simulink subsystem "PTI"  (R2025a)
settings: Solver=VariableStepAuto  StartTime=0.0  StopTime=10.0  RelTol=1e-3
libraries: px4Utilslib x22
settings Model: Creator=gurt1  LastModifiedBy=gurt1

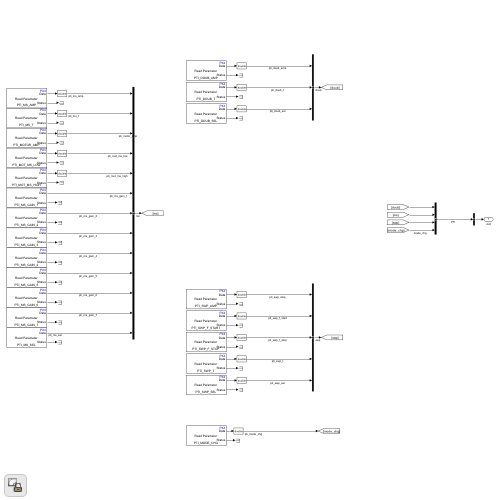
[thumbnail: Simulink's stored preview of the top-level diagram]
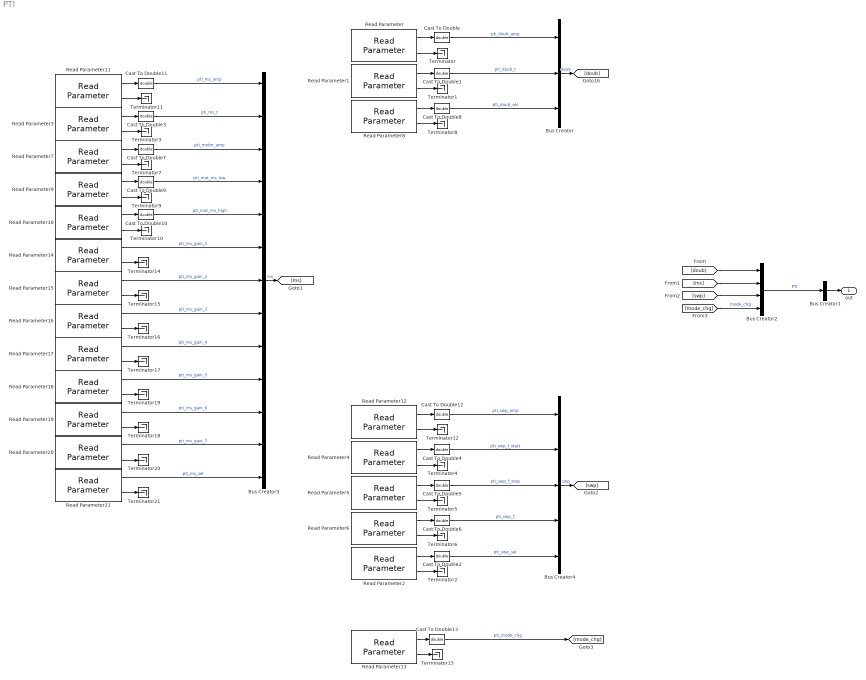
== system PTI ==
  Bus Creator : BusCreator  Inputs=3
  Bus Creator1 : BusCreator  Inputs=1
  Bus Creator2 : BusCreator  Inputs=4
  Bus Creator3 : BusCreator  Inputs=13
  Bus Creator4 : BusCreator  Inputs=5
  Cast To Double{,1..13} (14 alike) : DataTypeConversion  OutDataTypeStr=double  SaturateOnIntegerOverflow=off  RndMeth=Floor
  Read Parameter : px4Utilslib/Read Parameter  ParameterName=PTI_DOUB_AMP  DataType=FLOAT  SampleTime=-1
  Read Parameter1 : px4Utilslib/Read Parameter  ParameterName=PTI_DOUB_T  DataType=FLOAT  SampleTime=-1
  Read Parameter10 : px4Utilslib/Read Parameter  ParameterName=PTI_MOT_MS_HIGH  DataType=FLOAT  SampleTime=-1
  Read Parameter11 : px4Utilslib/Read Parameter  ParameterName=PTI_MS_AMP  DataType=FLOAT  SampleTime=-1
  Read Parameter12 : px4Utilslib/Read Parameter  ParameterName=PTI_SWP_AMP  DataType=FLOAT  SampleTime=-1
  Read Parameter13 : px4Utilslib/Read Parameter  ParameterName=PTI_MODE_CHG  DataType=FLOAT  SampleTime=-1
  Read Parameter14 : px4Utilslib/Read Parameter  ParameterName=PTI_MS_GAIN_1  DataType=FLOAT  SampleTime=-1
  Read Parameter15 : px4Utilslib/Read Parameter  ParameterName=PTI_MS_GAIN_2  DataType=FLOAT  SampleTime=-1
  Read Parameter16 : px4Utilslib/Read Parameter  ParameterName=PTI_MS_GAIN_3  DataType=FLOAT  SampleTime=-1
  Read Parameter17 : px4Utilslib/Read Parameter  ParameterName=PTI_MS_GAIN_4  DataType=FLOAT  SampleTime=-1
  Read Parameter18 : px4Utilslib/Read Parameter  ParameterName=PTI_MS_GAIN_5  DataType=FLOAT  SampleTime=-1
  Read Parameter19 : px4Utilslib/Read Parameter  ParameterName=PTI_MS_GAIN_6  DataType=FLOAT  SampleTime=-1
  Read Parameter2 : px4Utilslib/Read Parameter  ParameterName=PTI_SWP_SEL  DataType=FLOAT  SampleTime=-1
  Read Parameter20 : px4Utilslib/Read Parameter  ParameterName=PTI_MS_GAIN_7  DataType=FLOAT  SampleTime=-1
  Read Parameter21 : px4Utilslib/Read Parameter  ParameterName=PTI_MS_SEL  DataType=FLOAT  SampleTime=-1
  Read Parameter3 : px4Utilslib/Read Parameter  ParameterName=PTI_MS_T  DataType=FLOAT  SampleTime=-1
  Read Parameter4 : px4Utilslib/Read Parameter  ParameterName=PTI_SWP_F_START  DataType=FLOAT  SampleTime=-1
  Read Parameter5 : px4Utilslib/Read Parameter  ParameterName=PTI_SWP_F_STOP  DataType=FLOAT  SampleTime=-1
  Read Parameter6 : px4Utilslib/Read Parameter  ParameterName=PTI_SWP_T  DataType=FLOAT  SampleTime=-1
  Read Parameter7 : px4Utilslib/Read Parameter  ParameterName=PTI_MOTOR_AMP  DataType=FLOAT  SampleTime=-1
  Read Parameter8 : px4Utilslib/Read Parameter  ParameterName=PTI_DOUB_SEL  DataType=FLOAT  SampleTime=-1
  Read Parameter9 : px4Utilslib/Read Parameter  ParameterName=PTI_MOT_MS_LOW  DataType=FLOAT  SampleTime=-1
  Terminator{,1..21} (22 alike) : Terminator
  out : Outport
  wires:
  Read Parameter/2 -> Terminator/1
  Read Parameter/1 -> Cast To Double/1
  Cast To Double/1 -> Bus Creator/1  "pti_doub_amp"
  Bus Creator1/1 -> out/1
  Bus Creator2/1 -> Bus Creator1/1  "PTI"
  Read Parameter1/1 -> Cast To Double1/1
  Read Parameter1/2 -> Terminator1/1
  Cast To Double1/1 -> Bus Creator/2  "pti_doub_t"
  Read Parameter6/2 -> Terminator6/1
  Read Parameter5/2 -> Terminator5/1
  Read Parameter5/1 -> Cast To Double5/1
  Cast To Double6/1 -> Bus Creator4/4  "pti_swp_t"
  Read Parameter6/1 -> Cast To Double6/1
  Read Parameter4/2 -> Terminator4/1
  Read Parameter4/1 -> Cast To Double4/1
  Cast To Double5/1 -> Bus Creator4/3  "pti_swp_f_stop"
  Cast To Double4/1 -> Bus Creator4/2  "pti_swp_f_start"
  Cast To Double11/1 -> Bus Creator3/1  "pti_ms_amp"
  Cast To Double3/1 -> Bus Creator3/2  "pti_ms_t"
  Read Parameter3/2 -> Terminator3/1
  Read Parameter3/1 -> Cast To Double3/1
  Read Parameter11/1 -> Cast To Double11/1
  Read Parameter11/2 -> Terminator11/1
  Cast To Double8/1 -> Bus Creator/3  "pti_doub_sel"
  Read Parameter8/1 -> Cast To Double8/1
  Read Parameter8/2 -> Terminator8/1
  Bus Creator/1 -> [doub]  "doub"
  Bus Creator3/1 -> [ms]  "ms"
  Bus Creator4/1 -> [swp]  "swp"
  [doub] -> Bus Creator2/1
  [ms] -> Bus Creator2/2
  [swp] -> Bus Creator2/3
  Read Parameter12/1 -> Cast To Double12/1
  Read Parameter12/2 -> Terminator12/1
  Cast To Double12/1 -> Bus Creator4/1  "pti_swp_amp"
  Read Parameter13/2 -> Terminator13/1
  Read Parameter13/1 -> Cast To Double13/1
  Cast To Double13/1 -> [mode_chg]  "pti_mode_chg"
  [mode_chg] -> Bus Creator2/4  "mode_chg"
  Read Parameter2/1 -> Cast To Double2/1
  Read Parameter2/2 -> Terminator2/1
  Cast To Double2/1 -> Bus Creator4/5  "pti_swp_sel"
  Read Parameter7/1 -> Cast To Double7/1
  Read Parameter7/2 -> Terminator7/1
  Cast To Double7/1 -> Bus Creator3/3  "pti_motor_amp"
  Read Parameter9/2 -> Terminator9/1
  Read Parameter9/1 -> Cast To Double9/1
  Read Parameter10/1 -> Cast To Double10/1
  Read Parameter10/2 -> Terminator10/1
  Cast To Double9/1 -> Bus Creator3/4  "pti_mot_ms_low"
  Cast To Double10/1 -> Bus Creator3/5  "pti_mot_ms_high"
  Read Parameter14/2 -> Terminator14/1
  Read Parameter15/2 -> Terminator15/1
  Read Parameter16/2 -> Terminator16/1
  Read Parameter17/2 -> Terminator17/1
  Read Parameter18/1 -> Bus Creator3/10  "pti_ms_gain_5"
  Read Parameter18/2 -> Terminator19/1
  Read Parameter19/2 -> Terminator18/1
  Read Parameter20/2 -> Terminator20/1
  Read Parameter14/1 -> Bus Creator3/6  "pti_ms_gain_1"
  Read Parameter15/1 -> Bus Creator3/7  "pti_ms_gain_2"
  Read Parameter16/1 -> Bus Creator3/8  "pti_ms_gain_3"
  Read Parameter17/1 -> Bus Creator3/9  "pti_ms_gain_4"
  Read Parameter19/1 -> Bus Creator3/11  "pti_ms_gain_6"
  Read Parameter20/1 -> Bus Creator3/12  "pti_ms_gain_7"
  Read Parameter21/2 -> Terminator21/1
  Read Parameter21/1 -> Bus Creator3/13  "pti_ms_sel"
